simulink model "a2"  (R2022a)
settings: Solver=FixedStepAuto  StartTime=0.0  StopTime=inf  FixedStep=1e-3  RelTol=1e-3  EnableMultiTasking=on
undefined symbols (not defined in the file): A0, A1, D0, D1, D10, D11, D12, D13, D2, D3, D4, D5, D6, D7, D8, D9, PTA0, PTA1, PTA2, PTB2, PTB23, PTB3, PTB9, PTC16, PTC17, PTC2, PTC3, PTC4, PTD0, PTD1, PTD2, PTD3
libraries: frdmk64flib x21, etargetslib x20
settings Model: ExtModeTrigDuration=5  Creator=haotianxue  LastModifiedBy=yuexu
settings OptimizationCC: EnhancedBackFolding=on  PassReuseOutputArgsAs=Individual arguments  ZeroExternalMemoryAtStartup=off  ZeroInternalMemoryAtStartup=off  MaxStackSize=64  OptimizeBlockOrder=speed  DifferentSizesBufferReuse=on  OptimizationCustomize=off  EfficientTunableParamExpr=on
settings DebuggingCC: ParameterTunabilityLossMsg=error  UnconnectedInputMsg=warning  UnconnectedOutputMsg=warning  UnconnectedLineMsg=warning
settings HardwareCC: ProdBitPerPointer=32  ProdBitPerSizeT=32  ProdBitPerPtrDiffT=32  ProdLargestAtomicInteger=Long  ProdLargestAtomicFloat=Double  ProdWordSize=32  ProdHWDeviceType=ARM Compatible->ARM Cortex
settings SFSimCC: MATLABDynamicMemAlloc=off
settings RTWCC: SystemTargetFile=ert.tlc  HardwareBoard=NXP FRDM-K64F  TLCOptions="-aInlineSetEventsForThisBaseRateFcn=TLC_FALSE -aSuppressMultiTaskScheduler=TLC_FALSE  -aRateBasedStepFcn=0"  TemplateMakefile=ert_default_tmf  Toolchain=GNU Tools for ARM Embedded Processors  DLArmComputeVersion=19.05
settings CodeAppCC: ForceParamTrailComments=on  IgnoreCustomStorageClasses=off  OperatorAnnotations=on  SimulinkDataObjDesc=on  SFDataObjDesc=on  InsertBlockDesc=on
settings ERTTargetCC: ExtModeTransport=4  ExtModeMexFile=sendToCommService

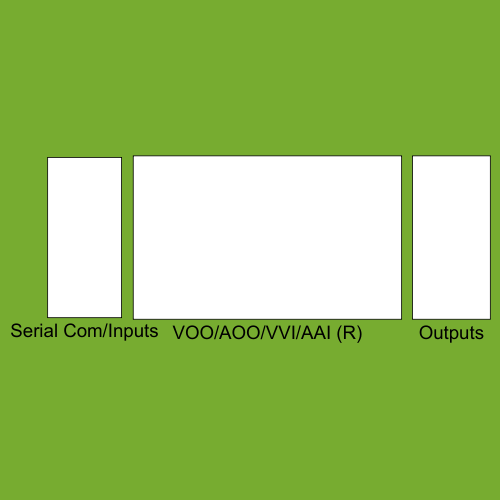
[thumbnail: Simulink's stored preview of the top-level diagram]
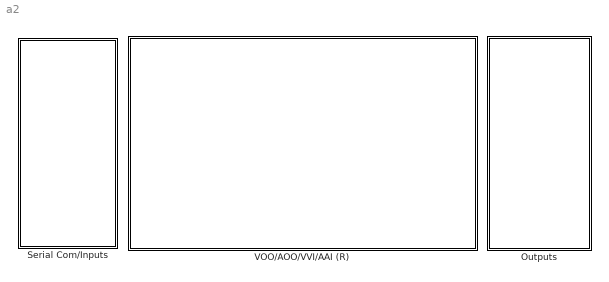
== system a2 ==
  Outputs : Subsystem
  Serial Com/Inputs : Subsystem
  VOO/AOO/VVI/AAI (R) : Subsystem

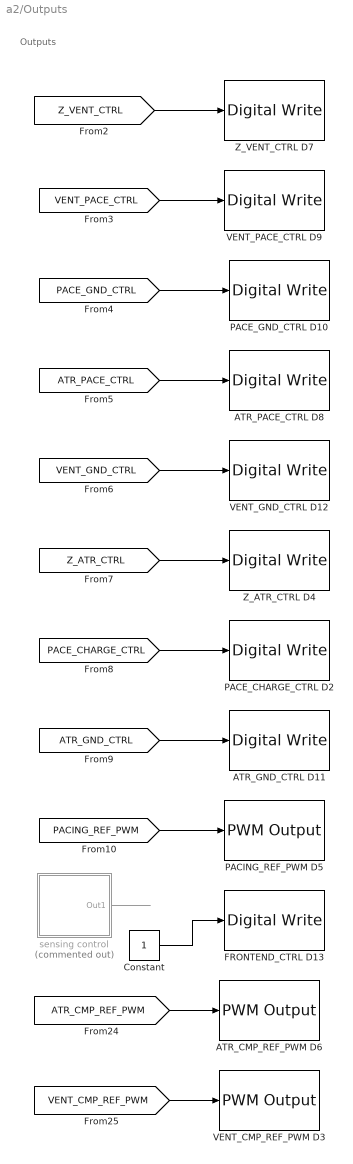
== system a2/Outputs ==
  note: Outputs
  ATR_CMP_REF_PWM D6 : frdmk64flib/PWM Output  Whichpin=PTC2 (D6)  InitialFrequency=2000  InitialDutyCycle=0
  ATR_GND_CTRL D11 : frdmk64flib/Digital Write  Whichpin=PTD2 (D11)
  ATR_PACE_CTRL D8 : frdmk64flib/Digital Write  Whichpin=PTA0 (D8)
  Constant : Constant
  FRONTEND_CTRL D13 : frdmk64flib/Digital Write  Whichpin=PTD1 (D13)
  PACE_CHARGE_CTRL D2 : frdmk64flib/Digital Write  Whichpin=PTB9 (D2)
  PACE_GND_CTRL D10 : frdmk64flib/Digital Write  Whichpin=PTD0 (D10)
  PACING_REF_PWM D5 : frdmk64flib/PWM Output  Whichpin=PTA2 (D5)  InitialFrequency=2000  InitialDutyCycle=0
  VENT_CMP_REF_PWM D3 : frdmk64flib/PWM Output  Whichpin=PTA1 (D3)  InitialFrequency=2000  InitialDutyCycle=0
  VENT_GND_CTRL D12 : frdmk64flib/Digital Write  Whichpin=PTD3 (D12)
  "VENT_PACE_CTRL D9  " : frdmk64flib/Digital Write  Whichpin=PTC4 (D9)
  Z_ATR_CTRL D4 : frdmk64flib/Digital Write  Whichpin=PTB23 (D4)
  Z_VENT_CTRL D7 : frdmk64flib/Digital Write  Whichpin=PTC3 (D7)
  sensing control : Subsystem  Commented=on
  wires:
  [VENT_GND_CTRL] -> VENT_GND_CTRL D12/1
  [ATR_PACE_CTRL] -> ATR_PACE_CTRL D8/1
  [PACE_CHARGE_CTRL] -> PACE_CHARGE_CTRL D2/1
  [VENT_PACE_CTRL] -> "VENT_PACE_CTRL D9  "/1
  [Z_VENT_CTRL] -> Z_VENT_CTRL D7/1
  [PACE_GND_CTRL] -> PACE_GND_CTRL D10/1
  [Z_ATR_CTRL] -> Z_ATR_CTRL D4/1
  [PACING_REF_PWM] -> PACING_REF_PWM D5/1
  [ATR_CMP_REF_PWM] -> ATR_CMP_REF_PWM D6/1
  [VENT_CMP_REF_PWM] -> VENT_CMP_REF_PWM D3/1
  [ATR_GND_CTRL] -> ATR_GND_CTRL D11/1
  sensing control/1(Out1) -> ?
  Constant/1 -> FRONTEND_CTRL D13/1

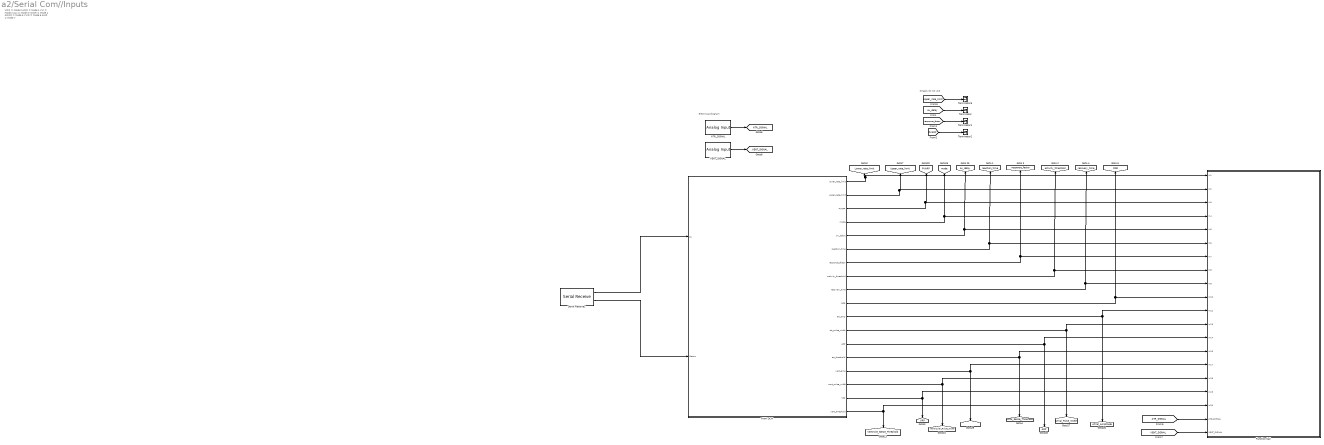
== system a2/Serial Com//Inputs ==
  note: Singals do not use
  note: VOO = Mode 0
      | AOO = Mode 1
      | VVI = Mode 2
      | AAI = Mode 3
      | VOOR = Mode 4
      | AOOR = Mode 5
      | VVIR = Mode 6
      | AAIR = Mode 7
  note: Electrocardiogram
  ATR_SIGNAL : frdmk64flib/Analog Input  Whichpin=PTB2 (A0)  SampleTime=-1
  From DCM : Stateflow chart  TreatAsAtomicUnit=on
  Function Call : Subsystem  TreatAsAtomicUnit=on
  Serial Receive1 : frdmk64flib/Serial Receive  SCIModule=0  Baudrate=uint32(9600)  Parity=None  StopBits=1  HardwareFlowControl=None  ByteOrder=LittleEndian  DataType=uint8  DataLength=74  BlockingMode=off  OutputStatus=on  SampleTime=-1
  Terminator{,1..2,5} (4 alike) : Terminator
  VENT_SIGNAL : frdmk64flib/Analog Input  Whichpin=PTB3 (A1)  SampleTime=-1
  tag scope: ARP=global, ATR_SIGNAL=global, Atrial_Amplitude=global, Atrial_Pulse_Width=global, Atrial_Sense_Threshold=global, Lower_rate_limit=global, MSR=global, PVARP=global, Upper_rate_limit=global, VENT_SIGNAL=global, VRP=global, Ventricle_Sense_Threshold=global, Ventricular_Amplitude=global, Ventricular_Pulse_Width=global, activity_threshold=global, av_delay=global, mode=global, reaction_time=global, recovery_time=global, response_factor=global
  wires:
  From DCM/10(MSR) -> [MSR], Function Call/10(In10)
  From DCM/18(vent_threshold) -> Function Call/18(In20), [Ventricle_Sense_Threshold]
  From DCM/17(VRP) -> Function Call/17(In19), [VRP]
  From DCM/14(atr_threshold) -> Function Call/14(In15), [Atrial_Sense_Threshold]
  From DCM/13(ARP) -> Function Call/13(In14), [ARP]
  From DCM/16(vent_pulse_width) -> Function Call/16(In18), [Ventricular_Pulse_Width]
  From DCM/3(PVARP) -> [PVARP], Function Call/3(In3)
  From DCM/12(atr_pulse_width) -> Function Call/12(In13), [Atrial_Pulse_Width]
  From DCM/7(response_factor) -> [response_factor], Function Call/7(In7)
  From DCM/9(recovery_time) -> [recovery_time], Function Call/9(In9)
  Serial Receive1/1 -> From DCM/1(Rx)
  From DCM/11(atr_amp) -> [Atrial_Amplitude], Function Call/11(In12)
  From DCM/5(av_delay) -> [av_delay], Function Call/5(In5)
  From DCM/15(vent_amp) -> Function Call/15(In17), [Ventricular_Amplitude]
  From DCM/6(reaction_time) -> [reaction_time], Function Call/6(In6)
  From DCM/8(activity_threshold) -> [activity_threshold], Function Call/8(In8)
  From DCM/4(mode) -> [mode], Function Call/4(In4)
  Serial Receive1/2 -> From DCM/2(Status)
  From DCM/2(upper_rate_limit) -> [Upper_rate_limit], Function Call/2(In2)
  From DCM/1(lower_rate_limit) -> [Lower_rate_limit], Function Call/1(In1)
  ATR_SIGNAL/1 -> [ATR_SIGNAL]
  VENT_SIGNAL/1 -> [VENT_SIGNAL]
  [av_delay] -> Terminator/1
  [response_factor] -> Terminator1/1
  [PVARP] -> Terminator2/1
  [Upper_rate_limit] -> Terminator5/1
  [ATR_SIGNAL] -> Function Call/19(ATR_SIGNAL)
  [VENT_SIGNAL] -> Function Call/20(VENT_SIGNAL)

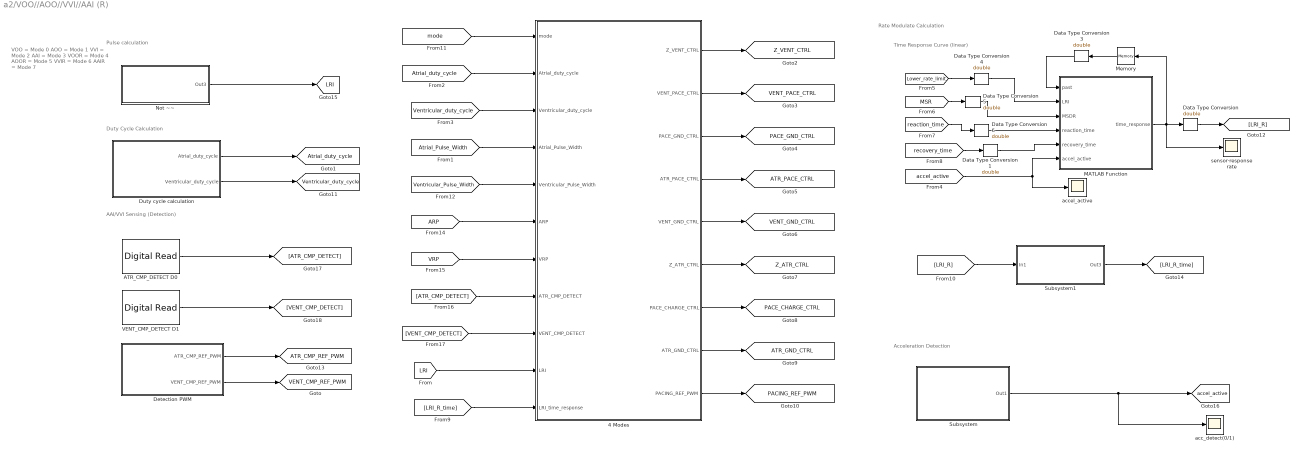
== system a2/VOO//AOO//VVI//AAI (R) ==
  note: Acceleration Detection
  note: Time Response Curve (linear)
  note: Rate Modulate Calculation
  note: Duty Cycle Calculation
  note: Pulse calculation
  note: AAI/VVI Sensing (Detection)
  note: VOO = Mode 0
      | AOO = Mode 1
      | VVI = Mode 2
      | AAI = Mode 3
      | VOOR = Mode 4
      | AOOR = Mode 5
      | VVIR = Mode 6
      | AAIR = Mode 7
  4 Modes : Stateflow chart  TreatAsAtomicUnit=on
      settings: PortSchema="{\"entries\":[{\"content\":{\"sides\":[{\"content\":{\"connectorIds\":[\"In1\",\"In2\",\"In3\",\"In4\",\"In5\",\"In6\",\"In7\",\"In8\",\"In10\",\"In9\",\"In11\"]},\"type\":\"ConnectorPlacement.EquallySpacedRectSide\",\"uuid\":\"cda6f2b2-e06a-45ee-a605-83fcbb92a490\"},{\"content\":{\"connectorIds\":[\"Out1\",\"Out2\",\"Out3\",\"Out4\",\"Out5\",\"Out6\",\"Out7\",\"Out8\",\"Out9\"],\"side\":\"RIGHT\"},\"type\":\"ConnectorPlacement.EquallySpacedRectSide\",\"uuid\":\"bbaec7b2-cf34-4072-a5a1-e7338d619e1a\"},{\"content\":{\"connectorIds\":[],\"side\":\"TOP\"},\"type\":\"ConnectorPlacement.EquallySpacedRectSide\",\"uuid\":\"0d445168-f6f3-41dc-a420-b501484e0774\"}]},\"type\":\"ConnectorPlacement.EquallySpacedConnector\",\"uuid\":\"5da4eaab-cd7d-4de3-80b7-75ac7c893a27\"}],\"packageUris\":[\"http://schema.mathworks.com/mf0/Connector/R2020b\"],\"version\":\"1.0\"}"
  ATR_CMP_DETECT D0 : frdmk64flib/Digital Read  Whichpin=PTC16 (D0)  SampleTime=-1
  Data Type Conversion{,1,3..6} (6 alike) : DataTypeConversion  OutDataTypeStr=double  SaturateOnIntegerOverflow=off  RndMeth=Floor
  Detection PWM : Subsystem
  Duty cycle calculation : Subsystem
  MATLAB Function : MATLAB Function  TreatAsAtomicUnit=on
  Memory : Memory
  Not ~~ : Subsystem
  Subsystem : Subsystem
  Subsystem1 : Subsystem
  VENT_CMP_DETECT D1 : frdmk64flib/Digital Read  Whichpin=PTC17 (D1)  SampleTime=-1
  acc_detect(0/1) : Scope
  accel_active : Scope
  sensor-response rate : Scope
  tag scope: ATR_CMP_REF_PWM=global, ATR_GND_CTRL=global, ATR_PACE_CTRL=global, Atrial_duty_cycle=global, LRI=global, PACE_CHARGE_CTRL=global, PACE_GND_CTRL=global, PACING_REF_PWM=global, VENT_CMP_REF_PWM=global, VENT_GND_CTRL=global, VENT_PACE_CTRL=global, Ventricular_duty_cycle=global, Z_ATR_CTRL=global, Z_VENT_CTRL=global, accel_active=global
  wires:
  4 Modes/5(VENT_GND_CTRL) -> [VENT_GND_CTRL]
  4 Modes/1(Z_VENT_CTRL) -> [Z_VENT_CTRL]
  4 Modes/8(ATR_GND_CTRL) -> [ATR_GND_CTRL]
  Detection PWM/1(ATR_CMP_REF_PWM) -> [ATR_CMP_REF_PWM]
  [mode] -> 4 Modes/1(mode)
  4 Modes/6(Z_ATR_CTRL) -> [Z_ATR_CTRL]
  4 Modes/3(PACE_GND_CTRL) -> [PACE_GND_CTRL]
  4 Modes/9(PACING_REF_PWM) -> [PACING_REF_PWM]
  [ATR_CMP_DETECT] -> 4 Modes/8(ATR_CMP_DETECT)
  4 Modes/2(VENT_PACE_CTRL) -> [VENT_PACE_CTRL]
  ATR_CMP_DETECT D0/1 -> [ATR_CMP_DETECT]
  [VENT_CMP_DETECT] -> 4 Modes/10(VENT_CMP_DETECT)
  [Atrial_Pulse_Width] -> 4 Modes/4(Atrial_Pulse_Width)
  [ARP] -> 4 Modes/6(ARP)
  [Ventricular_Pulse_Width] -> 4 Modes/5(Ventricular_Pulse_Width)
  4 Modes/4(ATR_PACE_CTRL) -> [ATR_PACE_CTRL]
  [VRP] -> 4 Modes/7(VRP)
  4 Modes/7(PACE_CHARGE_CTRL) -> [PACE_CHARGE_CTRL]
  Detection PWM/2(VENT_CMP_REF_PWM) -> [VENT_CMP_REF_PWM]
  Duty cycle calculation/1(Atrial_duty_cycle) -> [Atrial_duty_cycle]
  Duty cycle calculation/2(Ventricular_duty_cycle) -> [Ventricular_duty_cycle]
  [Atrial_duty_cycle] -> 4 Modes/2(Atrial_duty_cycle)
  [Ventricular_duty_cycle] -> 4 Modes/3(Ventricular_duty_cycle)
  VENT_CMP_DETECT D1/1 -> [VENT_CMP_DETECT]
  Not ~~/1(Out3) -> [LRI]
  [LRI] -> 4 Modes/9(LRI)
  [accel_active] -> accel_active/1, MATLAB Function/6(accel_active)
  [reaction_time] -> Data Type Conversion6/1
  MATLAB Function/1(time_response) -> Data Type Conversion/1, Memory/1, sensor-response rate/1
  Subsystem/1(Out1) -> acc_detect(0/1)/1, [accel_active]
  [LRI_R_time] -> 4 Modes/11(LRI_time_response)
  [Lower_rate_limit] -> Data Type Conversion4/1
  [MSR] -> Data Type Conversion5/1
  Data Type Conversion6/1 -> MATLAB Function/4(reaction_time)
  [recovery_time] -> Data Type Conversion1/1
  Data Type Conversion1/1 -> MATLAB Function/5(recovery_time)
  Data Type Conversion/1 -> [LRI_R]
  Memory/1 -> Data Type Conversion3/1
  Data Type Conversion3/1 -> MATLAB Function/1(past)
  Data Type Conversion4/1 -> MATLAB Function/2(LRI)
  Data Type Conversion5/1 -> MATLAB Function/3(MSDR)
  [LRI_R] -> Subsystem1/1(In1)
  Subsystem1/1(Out3) -> [LRI_R_time]

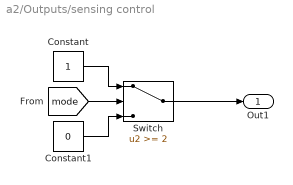
== system a2/Outputs/sensing control ==
  Constant : Constant
  Constant1 : Constant  Value=0
  Switch : Switch  Threshold=2  SaturateOnIntegerOverflow=off  InputSameDT=off
  Out1 : Outport
  wires:
  Constant/1 -> Switch/1
  Constant1/1 -> Switch/3
  [mode] -> Switch/2
  Switch/1 -> Out1/1

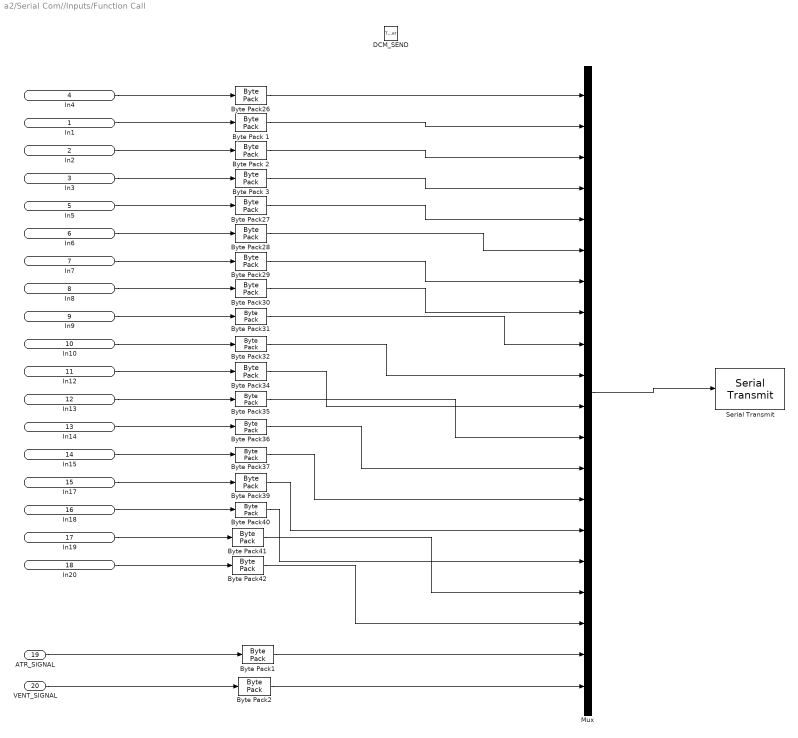
== system a2/Serial Com//Inputs/Function Call ==
  In1 : Inport
  In2 : Inport  Port=2
  In3 : Inport  Port=3
  In4 : Inport  Port=4
  In5 : Inport  Port=5
  In6 : Inport  Port=6
  In7 : Inport  Port=7
  In8 : Inport  Port=8
  In9 : Inport  Port=9
  In10 : Inport  Port=10
  In12 : Inport  Port=11
  In13 : Inport  Port=12
  In14 : Inport  Port=13
  In15 : Inport  Port=14
  In17 : Inport  Port=15
  In18 : Inport  Port=16
  In19 : Inport  Port=17
  In20 : Inport  Port=18
  ATR_SIGNAL : Inport  Port=19
  VENT_SIGNAL : Inport  Port=20
  DCM_SEND : TriggerPort  TriggerType=function-call  IsSimulinkFunction=on  FunctionName=DCM_SEND  VariantControl=Variant
  Byte Pack 1 : etargetslib/Byte Pack  datatypes={'uint8'}  byteAlign=1
  Byte Pack 2 : etargetslib/Byte Pack  datatypes={'uint8'}  byteAlign=1
  Byte Pack 3 : etargetslib/Byte Pack  datatypes={'uint16'}  byteAlign=1
  Byte Pack{1..2,30,34..35,37,39..40,42} (9 alike) : etargetslib/Byte Pack  datatypes={'double'}  byteAlign=1
  Byte Pack{26..27,29,32} (4 alike) : etargetslib/Byte Pack  datatypes={'uint8'}  byteAlign=1
  Byte Pack{28,31,36,41} (4 alike) : etargetslib/Byte Pack  datatypes={'uint16'}  byteAlign=1
  Mux : Mux  Inputs=20
  Serial Transmit : frdmk64flib/Serial Transmit  SCIModule=0  Baudrate=uint32(9600)  Parity=None  StopBits=1  HardwareFlowControl=None  ByteOrder=LittleEndian  BlockingMode=on  OutputStatus=on
  wires:
  In1/1 -> Byte Pack 1/1
  In2/1 -> Byte Pack 2/1
  In3/1 -> Byte Pack 3/1
  In4/1 -> Byte Pack26/1
  In5/1 -> Byte Pack27/1
  In6/1 -> Byte Pack28/1
  In7/1 -> Byte Pack29/1
  In8/1 -> Byte Pack30/1
  In9/1 -> Byte Pack31/1
  In10/1 -> Byte Pack32/1
  In12/1 -> Byte Pack34/1
  In13/1 -> Byte Pack35/1
  In14/1 -> Byte Pack36/1
  In15/1 -> Byte Pack37/1
  In17/1 -> Byte Pack39/1
  In18/1 -> Byte Pack40/1
  In19/1 -> Byte Pack41/1
  In20/1 -> Byte Pack42/1
  Byte Pack27/1 -> Mux/5
  Byte Pack28/1 -> Mux/6
  Byte Pack29/1 -> Mux/7
  Byte Pack30/1 -> Mux/8
  Byte Pack31/1 -> Mux/9
  Byte Pack32/1 -> Mux/10
  Byte Pack34/1 -> Mux/11
  Byte Pack35/1 -> Mux/12
  Byte Pack36/1 -> Mux/13
  Byte Pack37/1 -> Mux/14
  Mux/1 -> Serial Transmit/1
  Byte Pack26/1 -> Mux/1
  Byte Pack 1/1 -> Mux/2
  Byte Pack 2/1 -> Mux/3
  Byte Pack 3/1 -> Mux/4
  Byte Pack39/1 -> Mux/15
  Byte Pack40/1 -> Mux/16
  Byte Pack41/1 -> Mux/17
  Byte Pack42/1 -> Mux/18
  ATR_SIGNAL/1 -> Byte Pack1/1
  Byte Pack1/1 -> Mux/19
  VENT_SIGNAL/1 -> Byte Pack2/1
  Byte Pack2/1 -> Mux/20

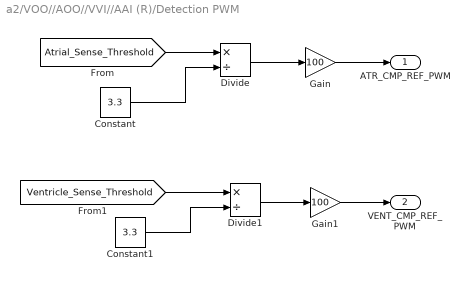
== system a2/VOO//AOO//VVI//AAI (R)/Detection PWM ==
  Constant : Constant  Value=3.3
  Constant1 : Constant  Value=3.3
  Divide : Product  Inputs=*/  RndMeth=Zero  SaturateOnIntegerOverflow=on
  Divide1 : Product  Inputs=*/  RndMeth=Zero  SaturateOnIntegerOverflow=on
  Gain : Gain  Gain=100
  Gain1 : Gain  Gain=100
  ATR_CMP_REF_PWM : Outport
  VENT_CMP_REF_PWM : Outport  Port=2
  wires:
  Divide/1 -> Gain/1
  Gain/1 -> ATR_CMP_REF_PWM/1
  Constant1/1 -> Divide1/2
  Divide1/1 -> Gain1/1
  Gain1/1 -> VENT_CMP_REF_PWM/1
  Constant/1 -> Divide/2
  [Atrial_Sense_Threshold] -> Divide/1
  [Ventricle_Sense_Threshold] -> Divide1/1

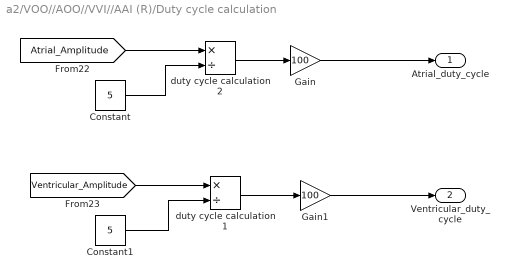
== system a2/VOO//AOO//VVI//AAI (R)/Duty cycle calculation ==
  Constant : Constant  Value=5
  Constant1 : Constant  Value=5
  Gain : Gain  Gain=100
  Gain1 : Gain  Gain=100
  duty cycle calculation1 : Product  Inputs=*/  RndMeth=Zero  SaturateOnIntegerOverflow=on
  duty cycle calculation2 : Product  Inputs=*/  RndMeth=Zero  SaturateOnIntegerOverflow=on
  Atrial_duty_cycle : Outport
  Ventricular_duty_cycle : Outport  Port=2
  wires:
  Gain/1 -> Atrial_duty_cycle/1
  Gain1/1 -> Ventricular_duty_cycle/1
  duty cycle calculation1/1 -> Gain1/1
  duty cycle calculation2/1 -> Gain/1
  Constant1/1 -> duty cycle calculation1/2
  Constant/1 -> duty cycle calculation2/2
  [Ventricular_Amplitude] -> duty cycle calculation1/1
  [Atrial_Amplitude] -> duty cycle calculation2/1

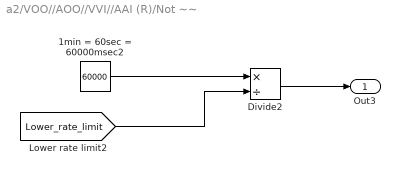
== system a2/VOO//AOO//VVI//AAI (R)/Not ~~ ==
  1min = 60sec = 60000msec2 : Constant  Value=60000
  Divide2 : Product  Inputs=*/
  Out3 : Outport
  wires:
  [Lower_rate_limit] -> Divide2/2
  1min = 60sec = 60000msec2/1 -> Divide2/1
  Divide2/1 -> Out3/1

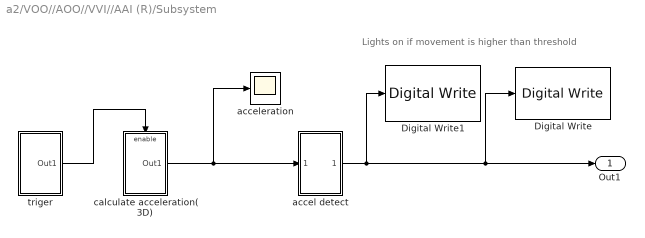
== system a2/VOO//AOO//VVI//AAI (R)/Subsystem ==
  note: Lights on if movement is higher than threshold
  Digital Write : frdmk64flib/Digital Write  Whichpin=GREEN_LED
  Digital Write1 : frdmk64flib/Digital Write  Whichpin=BLUE_LED
  accel detect : Subsystem
  acceleration : Scope
  calculate acceleration(3D) : Subsystem
  triger : Subsystem
  Out1 : Outport
  wires:
  calculate acceleration(3D)/1(Out1) -> acceleration/1, accel detect/1(In1)
  accel detect/1(Out1) -> Out1/1, Digital Write/1, Digital Write1/1
  triger/1(Out1) -> calculate acceleration(3D)/Enable

== system a2/VOO//AOO//VVI//AAI (R)/Subsystem1 ==
  In1 : Inport
  1min = 60sec = 60000msec2 : Constant  Value=60000
  Divide2 : Product  Inputs=*/
  Out3 : Outport
  wires:
  1min = 60sec = 60000msec2/1 -> Divide2/1
  Divide2/1 -> Out3/1
  In1/1 -> Divide2/2

== system a2/VOO//AOO//VVI//AAI (R)/Subsystem/accel detect ==
  In1 : Inport
  Relational Operator : RelationalOperator  OutDataTypeStr=boolean  RndMeth=Simplest  InputSameDT=off
  Out1 : Outport
  wires:
  [activity_threshold] -> Relational Operator/2
  In1/1 -> Relational Operator/1
  Relational Operator/1 -> Out1/1

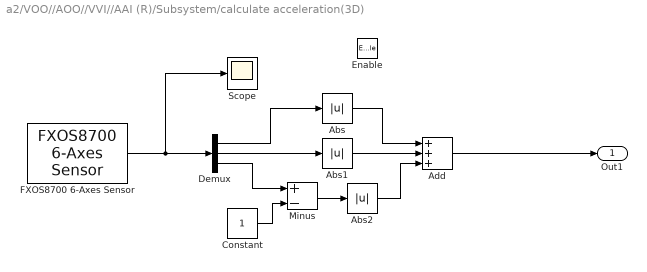
== system a2/VOO//AOO//VVI//AAI (R)/Subsystem/calculate acceleration(3D) ==
  Enable : EnablePort
  Abs : Abs  SaturateOnIntegerOverflow=off
  Abs1 : Abs  SaturateOnIntegerOverflow=off
  Abs2 : Abs  SaturateOnIntegerOverflow=off
  Add : Sum  Inputs=+++
  Constant : Constant
  Demux : Demux  Outputs=3
  FXOS8700 6-Axes Sensor : frdmk64flib/FXOS8700 6-Axes Sensor  Activesensor=Accelerometer only  ODR=100Hz  HybridODR=400Hz  Accelfullrange=-4g to +4g  SampleTime=-1
  Minus : Sum  Inputs=+-
  Scope : Scope
  Out1 : Outport
  wires:
  Abs1/1 -> Add/2
  Abs2/1 -> Add/3
  Demux/1 -> Abs/1
  FXOS8700 6-Axes Sensor/1 -> Scope/1, Demux/1
  Abs/1 -> Add/1
  Minus/1 -> Abs2/1
  Demux/2 -> Abs1/1
  Demux/3 -> Minus/1
  Constant/1 -> Minus/2
  Add/1 -> Out1/1

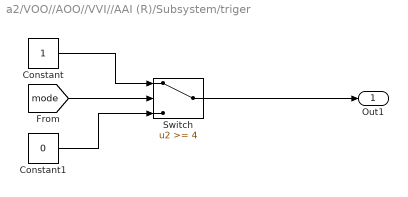
== system a2/VOO//AOO//VVI//AAI (R)/Subsystem/triger ==
  Constant : Constant
  Constant1 : Constant  Value=0
  Switch : Switch  Threshold=4  SaturateOnIntegerOverflow=off  InputSameDT=off
  Out1 : Outport
  wires:
  Constant/1 -> Switch/1
  [mode] -> Switch/2
  Constant1/1 -> Switch/3
  Switch/1 -> Out1/1

== stateflow chart a2/Serial Com//Inputs/From DCM ==
  state Default
    %Setting values to variables if
    %not initialized in DCM
    entry:
    %GENERAL
    mode = 0;
    lower_rate_limit = 60;
    upper_rate_limit = 120;
    PVARP = 200;
    av_delay=150;
    reaction_time = 10;
    response_factor = 16;
    activity_threshold = 2.3;
    recovery_time = 20;
    MSR = 180;
    %ATRIUM
    atr_amp = 3.5;
    atr_pulse_width = 10;
    ARP = 175;
    atr_threshold = 1.8;
    %VENTRICLE
    vent_amp = 3.5;
    vent_pulse_width = 10;
    VRP = 176;
    vent_threshold = 2.2;
  state SET_PARAM
    entry:
    mode = Rx(3);
    lower_rate_limit = Rx(4);
    upper_rate_limit = Rx(5);
    PVARP = typecast(Rx(6:7), 'uint16');
    av_delay = Rx(8);
    reaction_time = typecast(Rx(9:10), 'uint16');
    response_factor = Rx(11);
    activity_threshold = typecast(Rx(12:19), 'double');
    recovery_time = typecast(Rx(20:21), 'uint16');
    MSR = Rx(22);
    %ATR
    atr_amp = typecast(Rx(23:30), 'double');
    atr_pulse_width = typecast(Rx(31:38), 'double');
    ARP = typecast(Rx(39:40), 'uint16');
    atr_threshold = typecast(Rx(41:48), 'double');
    %VENT
    vent_amp = typecast(Rx(49:56), 'double');
    vent_pulse_width = typecast(Rx(57:64), 'double');
    VRP = typecast(Rx(65:66),'uint16');
    vent_threshold = typecast(Rx(67:74), 'double');
  state STANDBY
  state ECHO_PARAM
    entry:
    DCM_SEND();
  (default) -> Default
  SET_PARAM -> STANDBY
  (junction 56) -> STANDBY [order 2]
  Default -> STANDBY
  STANDBY -> (junction 56) : [Status == 0]
  (junction 56) -> (junction 62) [order 1] : [Rx(1) == hex2dec('16')]
  (junction 62) -> SET_PARAM [order 1] : [Rx(2) == hex2dec('55')]
  (junction 62) -> ECHO_PARAM [order 2] : [Rx(2) == hex2dec('22')]
  ECHO_PARAM -> STANDBY
  data: Rx input uint8; Status input uint8; lower_rate_limit output uint8; upper_rate_limit output uint8; PVARP output uint16; mode output uint8; av_delay output uint8; reaction_time output uint16; response_factor output uint8; activity_threshold output double; recovery_time output uint16; MSR output uint8; atr_amp output double; atr_pulse_width output double; ARP output uint16; atr_threshold output double; vent_amp output double; vent_pulse_width output double; VRP output uint16; vent_threshold output double

== stateflow chart a2/VOO//AOO//VVI//AAI (R)/4 Modes ==
  state VOOR
    state VOOR [group]
      state Charging
        entry:
        %Charging C22
        ATR_PACE_CTRL = LOW
        VENT_PACE_CTRL = LOW
        PACING_REF_PWM = Ventricular_duty_cycle
        PACE_CHARGE_CTRL = HIGH
        %Discharging Blocking Cap C21
        PACE_GND_CTRL = HIGH
        VENT_PACE_CTRL = LOW
        Z_ATR_CTRL = LOW
        Z_VENT_CTRL = LOW
        ATR_PACE_CTRL = LOW
        ATR_GND_CTRL = LOW
        VENT_GND_CTRL = HIGH
      state Pacing
        entry:
        %Discharge C22 (Charge C21)
        PACE_CHARGE_CTRL = LOW
        PACE_GND_CTRL = HIGH
        ATR_PACE_CTRL = LOW
        ATR_GND_CTRL = LOW
        Z_ATR_CTRL = LOW
        Z_VENT_CTRL = LOW
        VENT_GND_CTRL = LOW
        VENT_PACE_CTRL = HIGH
      VOOR.VOOR.Charging -> VOOR.VOOR.Pacing [order 2] : [after(0.5*LRI_time_response-Ventricular_Pulse_Width,msec)]
      VOOR.VOOR.Pacing -> VOOR.VOOR.Charging : [after(Ventricular_Pulse_Width,msec)]
  state AOOR
    state AOOR [group]
      state Charging
        entry:
        %Charging C22
        ATR_PACE_CTRL = LOW
        VENT_PACE_CTRL = LOW
        PACING_REF_PWM = Atrial_duty_cycle
        PACE_CHARGE_CTRL = HIGH
        %Discharging Blocking Cap C21
        PACE_GND_CTRL = HIGH
        VENT_PACE_CTRL = LOW
        Z_ATR_CTRL = LOW
        Z_VENT_CTRL = LOW
        ATR_PACE_CTRL = LOW
        ATR_GND_CTRL = HIGH
        VENT_GND_CTRL = LOW
      state Pacing
        entry:
        %Discharge C22 (Charge C21)
        PACE_CHARGE_CTRL = LOW
        PACE_GND_CTRL = HIGH
        ATR_PACE_CTRL = HIGH
        ATR_GND_CTRL = LOW
        Z_ATR_CTRL = LOW
        Z_VENT_CTRL = LOW
        VENT_GND_CTRL = LOW
        VENT_PACE_CTRL = LOW
      AOOR.AOOR.Charging -> AOOR.AOOR.Pacing [order 1] : after(0.5*LRI_time_response-Atrial_Pulse_Width,msec)
      AOOR.AOOR.Pacing -> AOOR.AOOR.Charging : after(Atrial_Pulse_Width,msec)
  state VVIR
    state VVIR [group]
      state Pacing
        entry:
        %Discharge C22 (Charge C21)
        PACE_CHARGE_CTRL = LOW
        PACE_GND_CTRL = HIGH
        ATR_PACE_CTRL = LOW
        ATR_GND_CTRL = LOW
        Z_ATR_CTRL = LOW
        Z_VENT_CTRL = LOW
        VENT_GND_CTRL = LOW
        VENT_PACE_CTRL = HIGH
      state Charging
        entry:
        %Charging C22
        ATR_PACE_CTRL = LOW
        VENT_PACE_CTRL = LOW
        PACING_REF_PWM = Ventricular_duty_cycle
        PACE_CHARGE_CTRL = HIGH
        %Discharging Blocking Cap C21
        PACE_GND_CTRL = HIGH
        VENT_PACE_CTRL = LOW
        Z_ATR_CTRL = LOW
        Z_VENT_CTRL = LOW
        ATR_PACE_CTRL = LOW
        ATR_GND_CTRL = LOW
        VENT_GND_CTRL = HIGH
      state VRP_Period
        %refactory period
      state Alert_Period
        %If nature pace occur
        %go back to VRP_Period
      VVIR.VVIR.Alert_Period -> VVIR.VVIR.VRP_Period [order 1] : [VENT_CMP_DETECT ==  true]
      VVIR.VVIR.VRP_Period -> VVIR.VVIR.Alert_Period : after(VRP, msec)
      VVIR.VVIR.Alert_Period -> VVIR.VVIR.Pacing [order 2] : after(0.5*LRI_time_response-Ventricular_Pulse_Width-VRP,msec)
      VVIR.VVIR.Charging -> VVIR.VVIR.Alert_Period [order 1] : after(VRP, msec)
      VVIR.VVIR.Pacing -> VVIR.VVIR.Charging : after(Ventricular_Pulse_Width,msec)
  state AAIR
    state AAIR [group]
      state Alert_Period
        %If nature pace occur
        %reset ARP_Period
      state ARP_Period
        %refractory period
      state Charging
        entry:
        %Charging C22
        ATR_PACE_CTRL = LOW
        VENT_PACE_CTRL = LOW
        PACING_REF_PWM = Atrial_duty_cycle
        PACE_CHARGE_CTRL = HIGH
        %Discharging Blocking Cap C21
        PACE_GND_CTRL = HIGH
        VENT_PACE_CTRL = LOW
        Z_ATR_CTRL = LOW
        Z_VENT_CTRL = LOW
        ATR_PACE_CTRL = LOW
        ATR_GND_CTRL = HIGH
        VENT_GND_CTRL = LOW
      state Pacing
        entry:
        %Discharge C22 (Charge C21)
        PACE_CHARGE_CTRL = LOW
        PACE_GND_CTRL = HIGH
        ATR_PACE_CTRL = HIGH
        ATR_GND_CTRL = LOW
        Z_ATR_CTRL = LOW
        Z_VENT_CTRL = LOW
        VENT_GND_CTRL = LOW
        VENT_PACE_CTRL = LOW
      AAIR.AAIR.Alert_Period -> AAIR.AAIR.ARP_Period [order 1] : [ATR_CMP_DETECT == true]
      AAIR.AAIR.Alert_Period -> AAIR.AAIR.Pacing [order 2] : after(0.5*LRI_time_response-Atrial_Pulse_Width-ARP, msec)
      AAIR.AAIR.ARP_Period -> AAIR.AAIR.Alert_Period : after(ARP, msec)
      AAIR.AAIR.Charging -> AAIR.AAIR.Alert_Period [order 1] : after(ARP, msec)
      AAIR.AAIR.Pacing -> AAIR.AAIR.Charging : after(Atrial_Pulse_Width, msec)
  state VOO
    state VOO [group]
      state Charging
        entry:
        %Charging C22
        ATR_PACE_CTRL = LOW
        VENT_PACE_CTRL = LOW
        PACING_REF_PWM = Ventricular_duty_cycle
        PACE_CHARGE_CTRL = HIGH
        %Discharging Blocking Cap C21
        PACE_GND_CTRL = HIGH
        VENT_PACE_CTRL = LOW
        Z_ATR_CTRL = LOW
        Z_VENT_CTRL = LOW
        ATR_PACE_CTRL = LOW
        ATR_GND_CTRL = LOW
        VENT_GND_CTRL = HIGH
      state Pacing
        entry:
        %Discharge C22 (Charge C21)
        PACE_CHARGE_CTRL = LOW
        PACE_GND_CTRL = HIGH
        ATR_PACE_CTRL = LOW
        ATR_GND_CTRL = LOW
        Z_ATR_CTRL = LOW
        Z_VENT_CTRL = LOW
        VENT_GND_CTRL = LOW
        VENT_PACE_CTRL = HIGH
      VOO.VOO.Charging -> VOO.VOO.Pacing [order 1] : [after(LRI-Ventricular_Pulse_Width,msec)]
      VOO.VOO.Pacing -> VOO.VOO.Charging : [after(Ventricular_Pulse_Width,msec)]
  state Start
    % mode 0 = VOO
    % mode 1 = AOO
    % mode 2 = VVI
    % mode 3 = AAI
    % mode 4 = VOOR
    % mode 5 = AOOR
    % mode 6 = VVIR
    % mode 7 = AAIR
  state AOO
    state AOO [group]
      state Charging
        entry:
        %Charging C22
        ATR_PACE_CTRL = LOW
        VENT_PACE_CTRL = LOW
        PACING_REF_PWM = Atrial_duty_cycle
        PACE_CHARGE_CTRL = HIGH
        %Discharging Blocking Cap C21
        PACE_GND_CTRL = HIGH
        VENT_PACE_CTRL = LOW
        Z_ATR_CTRL = LOW
        Z_VENT_CTRL = LOW
        ATR_PACE_CTRL = LOW
        ATR_GND_CTRL = HIGH
        VENT_GND_CTRL = LOW
      state Pacing
        entry:
        %Discharge C22 (Charge C21)
        PACE_CHARGE_CTRL = LOW
        PACE_GND_CTRL = HIGH
        ATR_PACE_CTRL = HIGH
        ATR_GND_CTRL = LOW
        Z_ATR_CTRL = LOW
        Z_VENT_CTRL = LOW
        VENT_GND_CTRL = LOW
        VENT_PACE_CTRL = LOW
      AOO.AOO.Charging -> AOO.AOO.Pacing [order 1] : after(LRI-Atrial_Pulse_Width,msec)
      AOO.AOO.Pacing -> AOO.AOO.Charging : after(Atrial_Pulse_Width,msec)
  state VVI
    state VVI [group]
      state Pacing
        entry:
        %Discharge C22 (Charge C21)
        PACE_CHARGE_CTRL = LOW
        PACE_GND_CTRL = HIGH
        ATR_PACE_CTRL = LOW
        ATR_GND_CTRL = LOW
        Z_ATR_CTRL = LOW
        Z_VENT_CTRL = LOW
        VENT_GND_CTRL = LOW
        VENT_PACE_CTRL = HIGH
      state Charging1
        entry:
        %Charging C22
        ATR_PACE_CTRL = LOW
        VENT_PACE_CTRL = LOW
        PACING_REF_PWM = Ventricular_duty_cycle
        PACE_CHARGE_CTRL = HIGH
        %Discharging Blocking Cap C21
        PACE_GND_CTRL = HIGH
        VENT_PACE_CTRL = LOW
        Z_ATR_CTRL = LOW
        Z_VENT_CTRL = LOW
        ATR_PACE_CTRL = LOW
        ATR_GND_CTRL = LOW
        VENT_GND_CTRL = HIGH
      state VRP_Period
        %refactory period
      state Alert_Period
        %If nature pace occur
        %go back to VRP_Period
      VVI.VVI.Alert_Period -> VVI.VVI.VRP_Period [order 1] : [VENT_CMP_DETECT ==  true]
      VVI.VVI.VRP_Period -> VVI.VVI.Alert_Period : after(VRP, msec)
      VVI.VVI.Alert_Period -> VVI.VVI.Pacing [order 2] : after(LRI-VRP,msec)
      Charging1 -> VVI.VVI.Alert_Period [order 1] : after(VRP, msec)
      VVI.VVI.Pacing -> Charging1 : after(Ventricular_Pulse_Width,msec)
  state AAI
    state AAI [group]
      state Alert_Period
        %If nature pace occur
        %reset ARP_Period
      state ARP_Period
        %refractory period
      state Charging
        entry:
        %Charging C22
        ATR_PACE_CTRL = LOW
        VENT_PACE_CTRL = LOW
        PACING_REF_PWM = Atrial_duty_cycle
        PACE_CHARGE_CTRL = HIGH
        %Discharging Blocking Cap C21
        PACE_GND_CTRL = HIGH
        VENT_PACE_CTRL = LOW
        Z_ATR_CTRL = LOW
        Z_VENT_CTRL = LOW
        ATR_PACE_CTRL = LOW
        ATR_GND_CTRL = HIGH
        VENT_GND_CTRL = LOW
      state Pacing
        entry:
        %Discharge C22 (Charge C21)
        PACE_CHARGE_CTRL = LOW
        PACE_GND_CTRL = HIGH
        ATR_PACE_CTRL = HIGH
        ATR_GND_CTRL = LOW
        Z_ATR_CTRL = LOW
        Z_VENT_CTRL = LOW
        VENT_GND_CTRL = LOW
        VENT_PACE_CTRL = LOW
      AAI.AAI.Alert_Period -> AAI.AAI.ARP_Period [order 1] : [ATR_CMP_DETECT == true]
      AAI.AAI.Alert_Period -> AAI.AAI.Pacing [order 2] : after(LRI - ARP, msec)
      AAI.AAI.ARP_Period -> AAI.AAI.Alert_Period : after(ARP, msec)
      AAI.AAI.Charging -> AAI.AAI.Alert_Period [order 1] : after(ARP, msec)
      AAI.AAI.Pacing -> AAI.AAI.Charging : after(Atrial_Pulse_Width, msec)
  (default) -> Start
  AOO.AOO.Charging -> Start [order 2] : [mode ~= 1]
  Charging1 -> Start [order 2] : [mode ~= 2]
  AAI.AAI.Charging -> Start [order 2] : [mode ~= 3]
  VOO.VOO.Charging -> Start [order 2] : [mode ~= 0]
  Start -> VOO.VOO.Charging [order 3] : [mode == 0]
  Start -> AOO.AOO.Charging [order 5] : [mode == 1]
  Start -> AAI.AAI.Charging [order 7] : [mode == 3]
  Start -> Charging1 [order 6] : [mode == 2]
  Start -> AAIR.AAIR.Charging [order 8] : [mode == 7]
  Start -> VOOR.VOOR.Charging [order 2] : [mode == 4 ]
  Start -> VVIR.VVIR.Charging [order 1] : [mode == 6]
  Start -> AOOR.AOOR.Charging [order 4] : [mode == 5]
  VOOR.VOOR.Charging -> Start [order 1] : [mode ~= 4]
  AAIR.AAIR.Charging -> Start [order 2] : [mode ~= 7]
  AOOR.AOOR.Charging -> Start [order 2] : [mode ~= 5]
  VVIR.VVIR.Charging -> Start [order 2] : [mode ~= 6]
  data: mode input; Z_VENT_CTRL output; VENT_PACE_CTRL output; PACE_GND_CTRL output; ATR_PACE_CTRL output; VENT_GND_CTRL output; Z_ATR_CTRL output; PACE_CHARGE_CTRL output; ATR_GND_CTRL output; PACING_REF_PWM output; LOW constant boolean =0; HIGH constant boolean =1; Atrial_duty_cycle input; Ventricular_duty_cycle input; Atrial_Pulse_Width input; Ventricular_Pulse_Width input; ARP input; VRP input; ATR_CMP_DETECT input; LRI input; VENT_CMP_DETECT input; LRI_time_response input

== matlab function a2/VOO//AOO//VVI//AAI (R)/MATLAB Function ==
  data: past input; LRI input; time_response output; MSDR input; reaction_time input; recovery_time input; accel_active input
function time_response = fcn(past, LRI, MSDR, reaction_time, recovery_time, accel_active)

%assuming all linear increase & decrease
pos_slope = (MSDR - LRI) / reaction_time;
neg_slope = -(MSDR - LRI) / recovery_time;

t_step = 1; %msec
if past == 0
    current = LRI;
else
    current = past;
end

%active
if accel_active == 1
    current = current + pos_slope*t_step;
    if current > MSDR
        current = MSDR;
    end

%disactive
else
    current = current + neg_slope*t_step;
    if current < LRI
        current = LRI;
    end
end

time_response=current;
